simulink model "AirConditioningFuzzyModel"  (R2013a)
settings: Solver=ode45  StartTime=0.0  StopTime=10.0  RelTol=1e-3
libraries: fuzblock x1
settings Model: Creator=zoza  LastModifiedBy=zoza

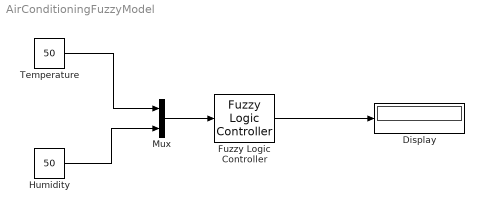
== system AirConditioningFuzzyModel ==
  Display : Display
  Fuzzy Logic Controller : fuzblock/Fuzzy Logic  Controller  fis=AirConditioningFuzzyControlMOD2
  Humidity : Constant  Value=50
  Mux : Mux  Inputs=2
  Temperature : Constant  Value=50
  wires:
  Temperature/1 -> Mux/1
  Humidity/1 -> Mux/2
  Mux/1 -> Fuzzy Logic Controller/1
  Fuzzy Logic Controller/1 -> Display/1
